simulink model "Practica1_ValeriaSinaiLaraRojas"  (R2025b)
settings: Solver=VariableStepAuto  StartTime=0.0  StopTime=10.0  RelTol=1e-3
settings Model: Creator=Cecilia  LastModifiedBy=Cecilia

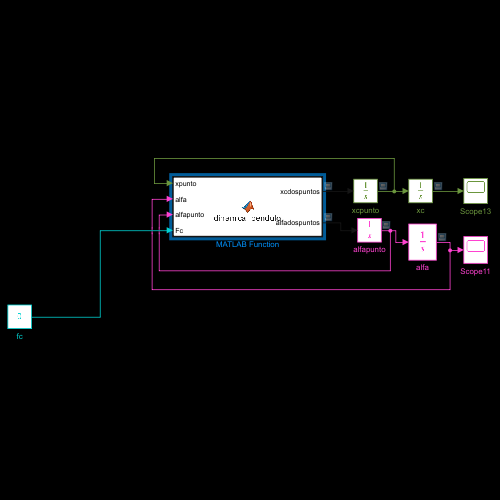
[thumbnail: Simulink's stored preview of the top-level diagram]
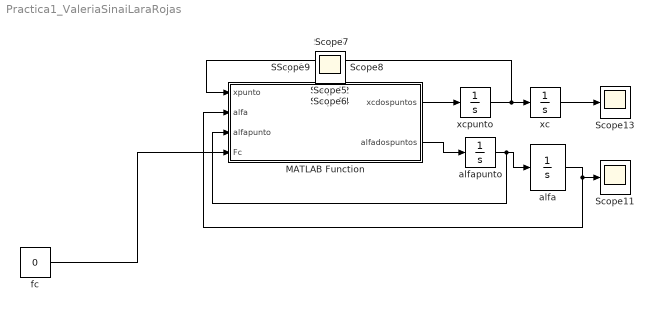
== system Practica1_ValeriaSinaiLaraRojas ==
  MATLAB Function : MATLAB Function  TreatAsAtomicUnit=on
  Scope{,1..14} (15 alike) : Scope
      Scope11 settings: ActiveDisplayYMinimum=-131.48407465072256  ActiveDisplayYMaximum=113.80126700389519  DataLoggingVariableName=ScopeData11
      Scope13 settings: ActiveDisplayYMinimum=-0.034445604585136014  ActiveDisplayYMaximum=0.18891055298295717  DataLoggingVariableName=ScopeData13
      Scope settings: ActiveDisplayYMinimum=-38.125251028573857  ActiveDisplayYMaximum=152.89151911182259
      Scope1 settings: ActiveDisplayYMinimum=-0.019299280698872393  ActiveDisplayYMaximum=0.17369352628985157
      Scope10 settings: ActiveDisplayYMinimum=-0.8226167636979  ActiveDisplayYMaximum=7.4035508732811026  DataLoggingVariableName=ScopeData10
      Scope12 settings: ActiveDisplayYMinimum=-0.0348137920991986  ActiveDisplayYMaximum=0.059476403971072976  DataLoggingVariableName=ScopeData12
      Scope14 settings: ActiveDisplayYMinimum=-0.43877220607816303  ActiveDisplayYMaximum=0.9911156204340954  DataLoggingVariableName=ScopeData14
      Scope2 settings: ActiveDisplayYMinimum=-1  ActiveDisplayYMaximum=1  DataLoggingVariableName=ScopeData2
      Scope3 settings: ActiveDisplayYMinimum=0.0074533000000000012  ActiveDisplayYMaximum=0.0274533  DataLoggingVariableName=ScopeData3
      Scope4 settings: ActiveDisplayYMinimum=-1  ActiveDisplayYMaximum=1  DataLoggingVariableName=ScopeData4
      Scope5 settings: ActiveDisplayYMinimum=-12.646349715905014  ActiveDisplayYMaximum=11.663775284094992  DataLoggingVariableName=ScopeData5
      Scope6 settings: ActiveDisplayYMinimum=-14.714328559045924  ActiveDisplayYMaximum=13.864228339058407  DataLoggingVariableName=ScopeData6
      Scope7 settings: ActiveDisplayYMinimum=-79.536633342529385  ActiveDisplayYMaximum=70.063728378599691  DataLoggingVariableName=ScopeData7
      Scope8 settings: ActiveDisplayYMinimum=-65.148438255906683  ActiveDisplayYMaximum=79.315647142098328  DataLoggingVariableName=ScopeData8
      Scope9 settings: ActiveDisplayYMinimum=-0.70786220385756682  ActiveDisplayYMaximum=2.7646509837927309  DataLoggingVariableName=ScopeData9
  alfa : Integrator  InitialCondition=0.01745
  alfapunto : Integrator
  fc : Constant  Value=0
  xc : Integrator
  xcpunto : Integrator
  wires:
  fc/1 -> MATLAB Function/4(Fc)
  xcpunto/1 -> MATLAB Function/1(xpunto), xc/1
  MATLAB Function/2(alfadospuntos) -> alfapunto/1
  alfapunto/1 -> MATLAB Function/3(alfapunto), alfa/1
  xc/1 -> Scope13/1
  MATLAB Function/1(xcdospuntos) -> xcpunto/1
  alfa/1 -> Scope11/1, MATLAB Function/2(alfa)

== matlab function Practica1_ValeriaSinaiLaraRojas/MATLAB Function ==
  data: xcdospuntos output; alfadospuntos output; xpunto input; alfa input; alfapunto input; Fc input
function [xcdospuntos, alfadospuntos]= dinamica_pendulo(xpunto, alfa, alfapunto, Fc)



Ip  = 0.0079;   % kg*m^2
Mc  = 0.7031;   % kg
Mp  = 0.23;     % kg
lp  = 0.3302;   % m
Beq = 4.3;      % N*s/m
Bp  = 0.0024;   % N*m*s/rad
g   = 9.81;     % m/s^2

D = (Mc + Mp)*Ip ...
  + Mc*Mp*lp^2 ...
  + Mp^2*lp^2*sin(alfa)^2;

xcdospuntos = ( ...
    (Ip + Mp*lp^2)*Fc ...
  + Mp^2*lp^2*g*cos(alfa)*sin(alfa) ...
  - (Ip + Mp*lp^2)*Beq*xpunto ...
  - (Ip*Mp*lp - Mp^2*lp^3)*alfapunto^2*sin(alfa) ...
  - Mp*lp*Bp*alfapunto*cos(alfa) ...
) / D;


alfadospuntos = ( ...
    (Mc + Mp)*Mp*g*lp*sin(alfa) ...
  - (Mc + Mp)*Bp*alfapunto ...
  + Fc*Mp*lp*cos(alfa) ...
  - Mp^2*lp^2*alfapunto^2*sin(alfa)*cos(alfa) ...
  - Beq*Mp*lp*xpunto*cos(alfa) ...
) / D;




end
